simulink model "upcount_test"  (R2016a)
settings: Solver=FixedStepDiscrete  SolverMode=SingleTasking  StartTime=0.0  StopTime=100  RelTol=1e-3
libraries: hdlsllib x1, lib_dsphdlcontrol_v1 x1
settings Model: DataTypeOverride=Off  Creator=mbabst  LastModifiedBy=mbabst
settings DataIOCC: SaveOutput=off  SaveTime=off
settings OptimizationCC: BlockReduction=off  ConditionallyExecuteInputs=off  DefaultParameterBehavior=Inlined
settings DebuggingCC: AlgebraicLoopMsg=error  SingleTaskRateTransMsg=error  StrictBusMsg=ErrorOnBusTreatedAsVector
settings HardwareCC: ProdBitPerPointer=32  ProdLargestAtomicFloat=None  ProdIntDivRoundTo=Undefined  ProdEndianess=Unspecified  ProdWordSize=32  ProdHWDeviceType=ASIC/FPGA->ASIC/FPGA  ProdEqTarget=off

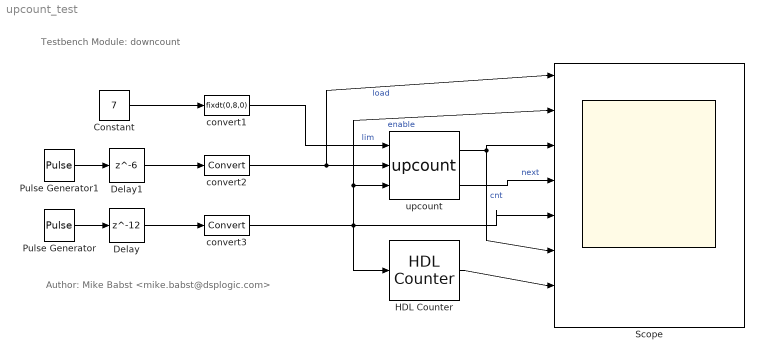
== system upcount_test ==
  note: Author: Mike Babst <mike.babst@dsplogic.com>
  note: Testbench
      | Module: downcount
  Constant : Constant  Value=7
  Delay : Delay  DelayLength=12  InitialCondition=0
  Delay1 : Delay  DelayLength=6  InitialCondition=0
  HDL Counter : hdlsllib/HDL Operations/HDL Counter  CountType=Count limited  CountInit=0  CountStep=1  CountMax=7  CountFromType=Initial value  CountFrom=0  CountResetPort=off  CountLoadPort=off  CountEnbPort=on  CountDirPort=off  CountDataType=Unsigned  CountWordLen=8  CountFracLen=0  CountSampTime=1
  Pulse Generator : DiscretePulseGenerator  Period=3
  Pulse Generator1 : DiscretePulseGenerator  Period=50  PhaseDelay=2
  Scope : Scope  NumInputPorts=8
  convert1 : DataTypeConversion  OutDataTypeStr=fixdt(0,8,0)
  convert2 : DataTypeConversion
  convert3 : DataTypeConversion
  upcount : lib_dsphdlcontrol_v1/upcount  FreeRun=off
  wires:
  Pulse Generator1/1 -> Delay1/1
  Pulse Generator/1 -> Delay/1
  Constant/1 -> convert1/1
  upcount/1 -> Scope/6, Scope/3  "cnt"
  upcount/2 -> Scope/4  "next"
  convert1/1 -> upcount/1  "lim"
  convert2/1 -> upcount/2, Scope/1  "load"
  Delay/1 -> convert3/1
  convert3/1 -> HDL Counter/1, Scope/5, upcount/3, Scope/2  "enable"
  Delay1/1 -> convert2/1
  HDL Counter/1 -> Scope/7
